simulink library "OSCILOS_SIM"  (R2014b)
settings: Solver=ode45  StartTime=0.0  StopTime=10.0  RelTol=1e-3
values from neighbouring files (symbols this model uses):
  c1 = sqrt(gamma * R * T1)    [parameters.m]
  c2 = sqrt(gamma * R * T2)    [parameters.m]
  dt = 10^-5    (= 1e-05)    [parameters.m]
  M11 = M(1,1)    [parameters.m]
  M12 = M(1,2)    [parameters.m]
  M13 = M(1,3)    [parameters.m]
  M21 = M(2,1)    [parameters.m]
  M22 = M(2,2)    [parameters.m]
  M23 = M(2,3)    [parameters.m]
  M31 = M(3,1)    [parameters.m]
  M32 = M(3,2)    [parameters.m]
  M33 = M(3,3)    [parameters.m]
  N1 = N(1)    [parameters.m]
  N2 = N(2)    [parameters.m]
  N3 = N(3)    [parameters.m]
  nphi = integral(fun, 0, alpha) / alpha    [jingxuan.m]    (also in parameters.m = 1)
  p1 = 101325    [parameters.m]
  Rd = (1 - 0.5 * (gamma - 1) * M2) / (1 + 0.5 * (gamma - 1) * M2)    [parameters.m]
  rho1 = p1 / (R * T1)    (= 1.20408475888)    [parameters.m]
  Rs = -((gamma * p2 / cp) * 0.5 * M2) / (1 + 0.5 * (gamma - 1) * M2)    [parameters.m]
  Ru = (1-gamma*M1+(gamma-1)*M1^2)/(1+gamma*M1+(gamma-1)*M1^2)    (= 0.734216975596)    [parameters.m]
  tau_1 = 0.01 / (2*pi)    (= 0.00159154943092)    [parameters.m]
  tau_d = 2 * xd / (c2 * (1 - M2^2))    [parameters.m]
  tau_f = 0.001    [parameters.m]
  tau_phi = 0.001    [parameters.m]
  tau_r1 = xr / (c2 - u2)    [parameters.m]
  tau_r2 = xr / (c2 + u2)    [parameters.m]
  tau_s = xd / (u2 * (1 - M2))    [parameters.m]
  tau_u = 2 * xu / (c1 * (1 - M1^2))    [parameters.m]
  u1 = M1 * c1    [parameters.m]
  u2 = (- b + sqrt(b^2 - 4 * a * c)) / (2 * a)    [parameters.m]
  xr = 0.5    [parameters.m]
  zc = 170    [parameters.m]
libraries: simulink x6, cstblocks x5
settings Model: Creator=Maxi  LastModifiedBy=Maxi

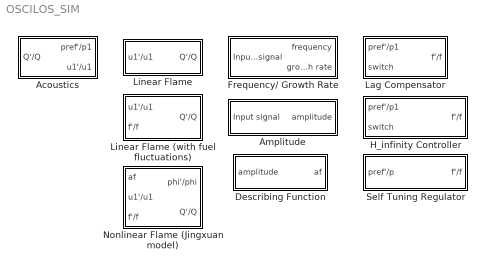
== system OSCILOS_SIM ==
  Acoustics : Subsystem
      mask Display:
      | %text(0.3,0.5,'Acoustics');
      | port_label('input', 1, 'Q''/Q');
      | port_label('output', 1, 'pref''/p1');
      | port_label('output', 2, 'u1''/u1');
  Amplitude : Subsystem
      mask Display: %text(0.3, 0.8, 'Amplitude')
  Describing Function : Subsystem
      mask Display: %text(0.15, 0.8, 'Describing function')
  Frequency/ Growth Rate : Subsystem
      mask Display: %text(0.1, 0.8, sprintf('Frequency/\nGrowth rate'))
  H_infinity Controller : Subsystem
      mask Display: text(0.4, 0.5, ' H_{ \infty }', 'texmode', 'on')
  Lag Compensator : Subsystem
      mask Display: %text(0.2, 0.53, 'Lag compensator')
  Linear Flame : Subsystem
      mask Display: %text(0.22,0.5,'Flame (linear)');
  Linear Flame (with fuel fluctuations) : Subsystem
      mask Display: %text(0.22,0.5,'Flame (linear)');
  Nonlinear Flame (Jingxuan model) : Subsystem
      mask Display: %text(0.3, 0.5, sprintf('Flame\n(Jingxuan)'))
  "Self Tuning Regulator " : Subsystem
      mask Display: text(0.4, 0.5, sprintf('STR'))

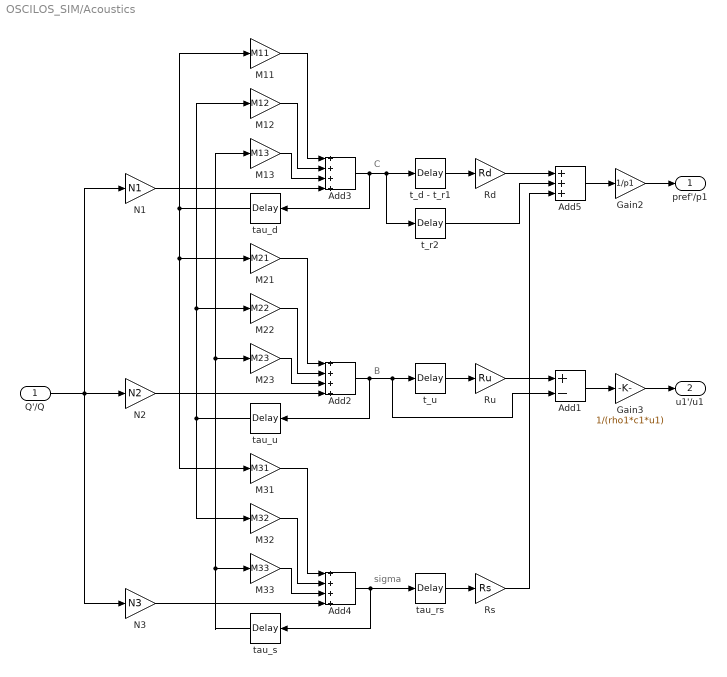
== system OSCILOS_SIM/Acoustics ==
  note: B
  note: C
  note: sigma
  Q'/Q : Inport
  Add1 : Sum  Inputs=+-
  Add2 : Sum  Inputs=++++
  Add3 : Sum  Inputs=++++
  Add4 : Sum  Inputs=++++
  Add5 : Sum  Inputs=+++
  Gain2 : Gain  Gain=1/p1
  Gain3 : Gain  Gain=1/(rho1*c1*u1)
  M11 : Gain  Gain=M11
  M12 : Gain  Gain=M12
  M13 : Gain  Gain=M13
  M21 : Gain  Gain=M21
  M22 : Gain  Gain=M22
  M23 : Gain  Gain=M23
  M31 : Gain  Gain=M31
  M32 : Gain  Gain=M32
  M33 : Gain  Gain=M33
  N1 : Gain  Gain=N1
  N2 : Gain  Gain=N2
  N3 : Gain  Gain=N3
  Rd : Gain  Gain=Rd
  Rs : Gain  Gain=Rs
  Ru : Gain  Gain=Ru
  t_d - t_r1 : TransportDelay  DelayTime=tau_d - tau_r1  BufferSize=4096
  t_r2 : TransportDelay  DelayTime=tau_r2  BufferSize=4096
  t_u : TransportDelay  DelayTime=tau_u  BufferSize=4096
  tau_d : TransportDelay  DelayTime=tau_d  BufferSize=4096
  tau_rs : TransportDelay  DelayTime=tau_s-xr/(c2-u2)  BufferSize=4096
  tau_s : TransportDelay  DelayTime=tau_s  BufferSize=4096
  tau_u : TransportDelay  DelayTime=tau_u  BufferSize=4096
  pref'/p1 : Outport
  u1'/u1 : Outport  Port=2
  wires:
  Ru/1 -> Add1/1
  t_u/1 -> Ru/1
  tau_d/1 -> M11/1, M21/1, M31/1
  tau_u/1 -> M32/1, M12/1, M22/1
  t_d - t_r1/1 -> Rd/1
  Rd/1 -> Add5/1
  t_r2/1 -> Add5/2
  Q'/Q/1 -> N3/1, N1/1, N2/1
  Add1/1 -> Gain3/1
  Add5/1 -> Gain2/1
  Gain2/1 -> pref'/p1/1
  Gain3/1 -> u1'/u1/1
  tau_s/1 -> M33/1, M13/1, M23/1
  N1/1 -> Add3/4
  M13/1 -> Add3/3
  M12/1 -> Add3/2
  M11/1 -> Add3/1
  N2/1 -> Add2/4
  M23/1 -> Add2/3
  M22/1 -> Add2/2
  M21/1 -> Add2/1
  N3/1 -> Add4/4
  M33/1 -> Add4/3
  M32/1 -> Add4/2
  M31/1 -> Add4/1
  Add3/1 -> tau_d/1, t_r2/1, t_d - t_r1/1
  Add2/1 -> Add1/2, t_u/1, tau_u/1
  tau_rs/1 -> Rs/1
  Add4/1 -> tau_rs/1, tau_s/1
  Rs/1 -> Add5/3

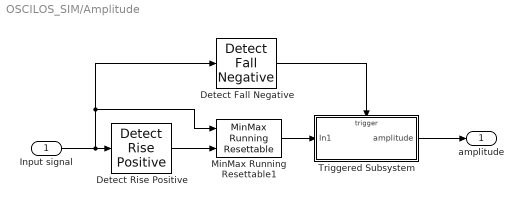
== system OSCILOS_SIM/Amplitude ==
  Input signal : Inport
  Detect Fall Negative : simulink/Logic and Bit Operations/Detect Fall Negative  vinit=0  InputProcessing=Inherited  OutDataTypeStr=boolean
  Detect Rise Positive : simulink/Logic and Bit Operations/Detect Rise Positive  vinit=0  InputProcessing=Inherited  OutDataTypeStr=boolean
  MinMax Running Resettable1 : simulink/Math Operations/MinMax Running Resettable  Function=max  vinit=0.0
  Triggered Subsystem : Subsystem  TreatAsAtomicUnit=on
  amplitude : Outport
  wires:
  Input signal/1 -> Detect Fall Negative/1, MinMax Running Resettable1/1, Detect Rise Positive/1
  Detect Rise Positive/1 -> MinMax Running Resettable1/2
  Detect Fall Negative/1 -> Triggered Subsystem/Trigger
  MinMax Running Resettable1/1 -> Triggered Subsystem/1(In1)
  Triggered Subsystem/1(amplitude) -> amplitude/1

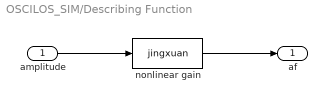
== system OSCILOS_SIM/Describing Function ==
  amplitude : Inport
  " nonlinear gain " : MATLABFcn  MATLABFcn=jingxuan
  af : Outport
  wires:
  amplitude/1 -> " nonlinear gain "/1
  " nonlinear gain "/1 -> af/1

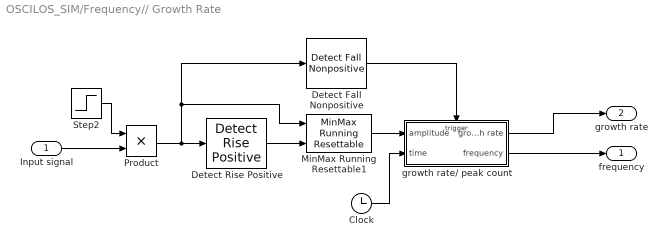
== system OSCILOS_SIM/Frequency// Growth Rate ==
  Input signal : Inport
  Clock : Clock
  Detect Fall Nonpositive : simulink/Logic and Bit Operations/Detect Fall Nonpositive  vinit=0  InputProcessing=Inherited  OutDataTypeStr=boolean
  Detect Rise Positive : simulink/Logic and Bit Operations/Detect Rise Positive  vinit=0  InputProcessing=Inherited  OutDataTypeStr=boolean
  MinMax Running Resettable1 : simulink/Math Operations/MinMax Running Resettable  Function=max  vinit=0.0
  Product : Product
  Step2 : Step  Time=0.05  SampleTime=0
  growth rate/ peak count : Subsystem  TreatAsAtomicUnit=on
  frequency : Outport
  growth rate : Outport  Port=2
  wires:
  Detect Rise Positive/1 -> MinMax Running Resettable1/2
  Detect Fall Nonpositive/1 -> growth rate/ peak count/Trigger
  MinMax Running Resettable1/1 -> growth rate/ peak count/1(amplitude)
  growth rate/ peak count/2(frequency) -> frequency/1
  Product/1 -> Detect Rise Positive/1, MinMax Running Resettable1/1, Detect Fall Nonpositive/1
  Step2/1 -> Product/1
  growth rate/ peak count/1(growth rate) -> growth rate/1
  Input signal/1 -> Product/2
  Clock/1 -> growth rate/ peak count/2(time)

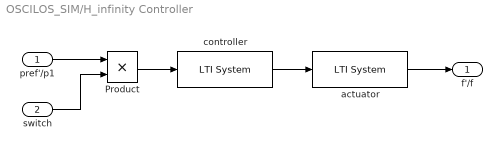
== system OSCILOS_SIM/H_infinity Controller ==
  pref'/p1 : Inport
  switch : Inport  Port=2
  Product : Product
  actuator : cstblocks/LTI System  sys=W_ac  IC=[]
  controller : cstblocks/LTI System  sys=Kinfinity  IC=[]
  f'/f : Outport
  wires:
  actuator/1 -> f'/f/1
  controller/1 -> actuator/1
  pref'/p1/1 -> Product/1
  Product/1 -> controller/1
  switch/1 -> Product/2

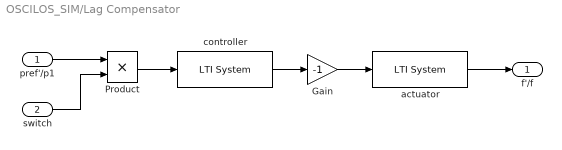
== system OSCILOS_SIM/Lag Compensator ==
  pref'/p1 : Inport
  switch : Inport  Port=2
  Gain : Gain  Gain=-1
  Product : Product
  actuator : cstblocks/LTI System  sys=W_ac  IC=[]
  controller : cstblocks/LTI System  sys=K_lag  IC=[]
  f'/f : Outport
  wires:
  actuator/1 -> f'/f/1
  controller/1 -> Gain/1
  pref'/p1/1 -> Product/1
  Product/1 -> controller/1
  switch/1 -> Product/2
  Gain/1 -> actuator/1

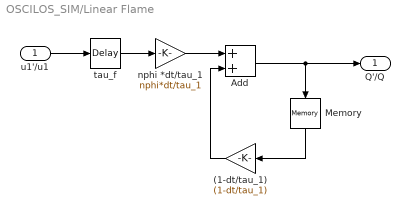
== system OSCILOS_SIM/Linear Flame ==
  u1'/u1 : Inport
  (1-dt/tau_1) : Gain  Gain=(1-dt/tau_1)
  Add : Sum
  Memory : Memory
  nphi *dt/tau_1 : Gain  Gain=nphi*dt/tau_1
  tau_f : TransportDelay  DelayTime=tau_f  BufferSize=4096
  Q'/Q : Outport
  wires:
  (1-dt/tau_1)/1 -> Add/2
  Memory/1 -> (1-dt/tau_1)/1
  Add/1 -> Q'/Q/1, Memory/1
  nphi *dt/tau_1/1 -> Add/1
  tau_f/1 -> nphi *dt/tau_1/1
  u1'/u1/1 -> tau_f/1

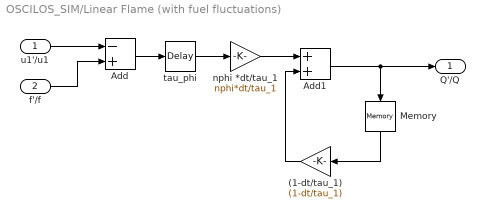
== system OSCILOS_SIM/Linear Flame (with fuel fluctuations) ==
  u1'/u1 : Inport
  f'/f : Inport  Port=2
  (1-dt/tau_1) : Gain  Gain=(1-dt/tau_1)
  Add : Sum  Inputs=-+
  Add1 : Sum
  Memory : Memory
  nphi *dt/tau_1 : Gain  Gain=nphi*dt/tau_1
  tau_phi : TransportDelay  DelayTime=tau_phi  BufferSize=4096
  Q'/Q : Outport
  wires:
  u1'/u1/1 -> Add/1
  f'/f/1 -> Add/2
  Add/1 -> tau_phi/1
  tau_phi/1 -> nphi *dt/tau_1/1
  nphi *dt/tau_1/1 -> Add1/1
  Add1/1 -> Memory/1, Q'/Q/1
  Memory/1 -> (1-dt/tau_1)/1
  (1-dt/tau_1)/1 -> Add1/2

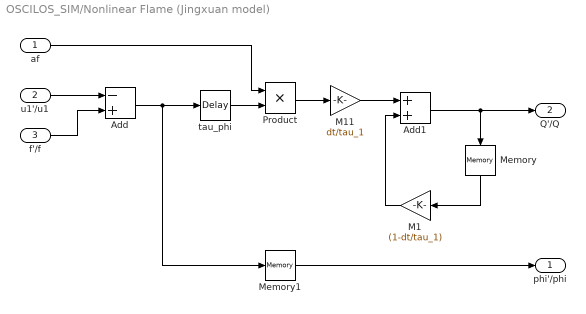
== system OSCILOS_SIM/Nonlinear Flame (Jingxuan model) ==
  af : Inport
  u1'/u1 : Inport  Port=2
  f'/f : Inport  Port=3
  Add : Sum  Inputs=-+
  Add1 : Sum
  M1 : Gain  Gain=(1-dt/tau_1)
  M11 : Gain  Gain=dt/tau_1
  Memory : Memory
  Memory1 : Memory
  Product : Product
  tau_phi : TransportDelay  DelayTime=tau_f  BufferSize=4096
  phi'/phi : Outport
  Q'/Q : Outport  Port=2
  wires:
  u1'/u1/1 -> Add/1
  f'/f/1 -> Add/2
  Add/1 -> Memory1/1, tau_phi/1
  M11/1 -> Add1/1
  Add1/1 -> Memory/1, Q'/Q/1
  Memory/1 -> M1/1
  M1/1 -> Add1/2
  tau_phi/1 -> Product/2
  af/1 -> Product/1
  Product/1 -> M11/1
  Memory1/1 -> phi'/phi/1

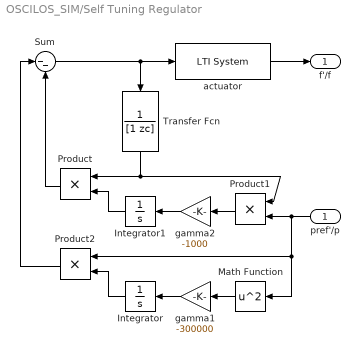
== system OSCILOS_SIM/Self Tuning Regulator  ==
  pref'/p : Inport
  Integrator : Integrator
  Integrator1 : Integrator
  Math Function : Math  Operator=square  SaturateOnIntegerOverflow=on
  Product : Product
  Product1 : Product
  Product2 : Product
  Sum : Sum  Inputs=|--
  Transfer Fcn : TransferFcn  Denominator=[1 zc]
  actuator : cstblocks/LTI System  sys=W_ac  IC=[]
  gamma1 : Gain  Gain=-300000
  gamma2 : Gain  Gain=-1000
  f'/f : Outport
  wires:
  actuator/1 -> f'/f/1
  Sum/1 -> actuator/1, Transfer Fcn/1
  Transfer Fcn/1 -> Product/1, Product1/1
  gamma2/1 -> Integrator1/1
  Product1/1 -> gamma2/1
  Integrator1/1 -> Product/2
  gamma1/1 -> Integrator/1
  Math Function/1 -> gamma1/1
  Integrator/1 -> Product2/2
  Product/1 -> Sum/2
  Product2/1 -> Sum/1
  pref'/p/1 -> Math Function/1, Product2/1, Product1/2

== system OSCILOS_SIM/Amplitude/Triggered Subsystem ==
  In1 : Inport
  Trigger : TriggerPort
  amplitude : Outport
  wires:
  In1/1 -> amplitude/1

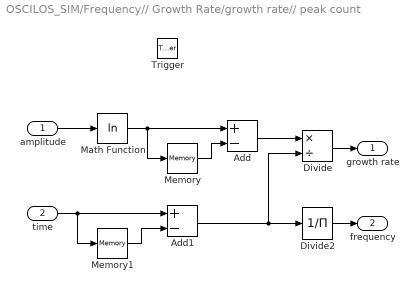
== system OSCILOS_SIM/Frequency// Growth Rate/growth rate// peak count ==
  amplitude : Inport
  time : Inport  Port=2
  Trigger : TriggerPort
  Add : Sum  Inputs=+-
  Add1 : Sum  Inputs=+-
  Divide : Product  Inputs=*/
  Divide2 : Product  Inputs=/
  Math Function : Math  Operator=log  SaturateOnIntegerOverflow=on
  Memory : Memory  InheritSampleTime=on
  Memory1 : Memory  InheritSampleTime=on
  growth rate : Outport
  frequency : Outport  Port=2
  wires:
  amplitude/1 -> Math Function/1
  Memory/1 -> Add/2
  time/1 -> Add1/1, Memory1/1
  Memory1/1 -> Add1/2
  Math Function/1 -> Memory/1, Add/1
  Add/1 -> Divide/1
  Add1/1 -> Divide2/1, Divide/2
  Divide/1 -> growth rate/1
  Divide2/1 -> frequency/1
